simulink model "harmonic_tracker"  (R2025b)
settings: Solver=VariableStepAuto  StartTime=0.0  StopTime=1  RelTol=1e-3
values from neighbouring files (symbols this model uses):
  Ad_fht2 = eye(2) + Afht1*ts_inv + 1/2*Afht1^2*ts_inv^2    [init_model.m]
  Ad_fht3 = expm(Afht1*ts_inv)    [init_model.m]
  Cfht1 = [1 0]    [init_model.m]
  delta_fht1 = 0.05    [init_model.m]
  Ld_fht1 = acker(Ad_fht1',Cfht1', polesd_fht1)    [init_model.m]
  Ld_fht2 = acker(Ad_fht2',Cfht1', polesd_fht1)    [init_model.m]
  Ld_fht3 = acker(Ad_fht3',Cfht1', polesd_fht1)    [init_model.m]
  omega_fht1 = 2*pi*frequency_set    (= 2513.27412287)    [init_model.m]
  ts_afe = 1/fPWM_AFE    (= 0.0001)    [init_model.m]
  ts_inv = 1/fPWM_INV    (= 0.0001)    [init_model.m]
libraries: sogi_quadrature_generator_ccaller x1
settings Model: SimulationMode=accelerator  Creator=ltnbda  LastModifiedBy=dbagn
settings SFSimCC: SimCustomHeaderCode=|
  | #include "first_harmonic_tracker_simulink.h"
  | #include "first_harmonic_tracker.h"
  | #include "sogi_flt_simulink.h"
  | #include "sogi_flt.h"
  | #include "harmonic_tracker_simulink.h"
  | #include "harmonic_tracker.h"
settings SFSimCC: SimUserSources=|
  | "first_harmonic_tracker_simulink.c"
  | "first_harmonic_tracker.c"
  | "sogi_flt_simulink.c"
  | "sogi_flt.c"
  | "harmonic_tracker_simulink.c"
  | "harmonic_tracker.c"
settings SFSimCC: SimUserIncludeDirs=|
  | include
  | src

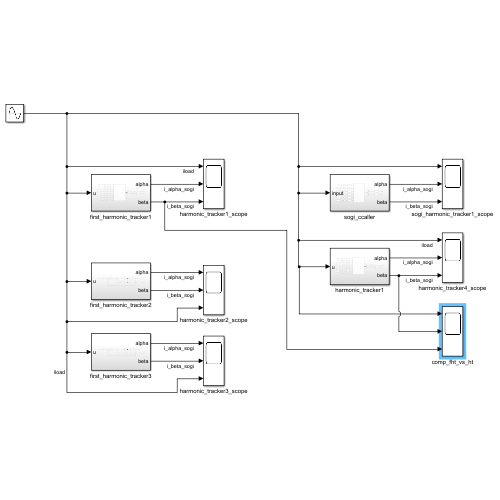
[thumbnail: Simulink's stored preview of the top-level diagram]
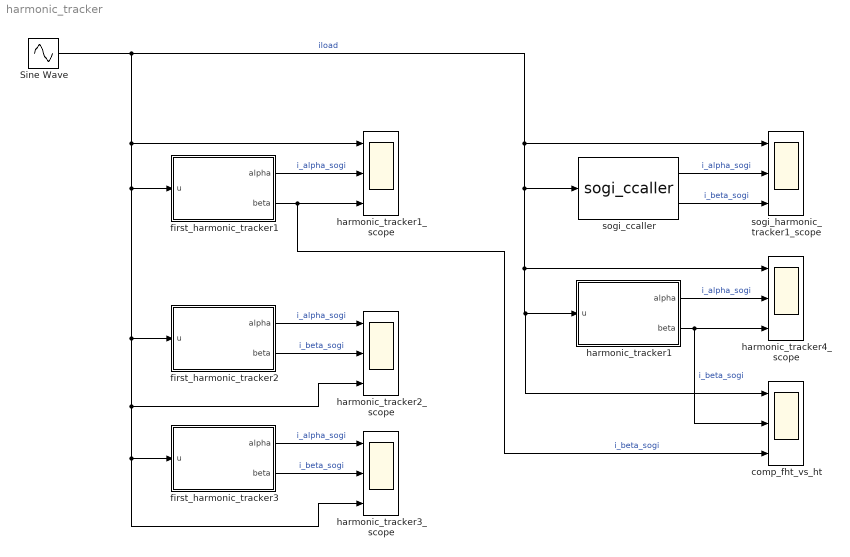
== system harmonic_tracker ==
  Sine Wave : Sin  Frequency=omega_fht1  SampleTime=0
  comp_fht_vs_ht : Scope  NumInputPorts=3
      settings: ActiveDisplayYMinimum=-1.6579339355230331  ActiveDisplayYMaximum=1.6235805600881577  DataLoggingVariableName=ScopeData5
  first_harmonic_tracker1 : Subsystem
  first_harmonic_tracker2 : Subsystem
  first_harmonic_tracker3 : Subsystem
  harmonic_tracker1 : Subsystem
  harmonic_tracker1_scope : Scope  NumInputPorts=3
      settings: ActiveDisplayYMinimum=-1.6579339355230331  ActiveDisplayYMaximum=1.6235805600881577
  harmonic_tracker2_scope : Scope  NumInputPorts=3
      settings: ActiveDisplayYMinimum=-1.2519895707446069  ActiveDisplayYMaximum=1.287638852418608
  harmonic_tracker3_scope : Scope  NumInputPorts=3
      settings: ActiveDisplayYMinimum=-1.251814205501226  ActiveDisplayYMaximum=1.2860605652281802  DataLoggingVariableName=ScopeData2
  harmonic_tracker4_scope : Scope  NumInputPorts=3
      settings: ActiveDisplayYMinimum=-1.6579339355230331  ActiveDisplayYMaximum=1.6235805600881577  DataLoggingVariableName=ScopeData4
  sogi_ccaller : sogi_quadrature_generator_ccaller/sogi_ccaller  SystemSampleTime=-1  VariantActivationTime=update diagram  EmptyChoice=off  PassThrough=off  PassThroughVariantControl=(default)  EmptyChoiceVariantControl=(default)  AllowFlexibleInterface=on  Latency=0  AutoFrameSizeCalculation=off
  sogi_harmonic_tracker1_scope : Scope  NumInputPorts=3
      settings: ActiveDisplayYMinimum=-1.4729834645986557  ActiveDisplayYMaximum=1.5802953094244003  DataLoggingVariableName=ScopeData3
  wires:
  first_harmonic_tracker1/1(alpha) -> harmonic_tracker1_scope/2  "i_alpha_sogi"
  first_harmonic_tracker1/2(beta) -> comp_fht_vs_ht/3, harmonic_tracker1_scope/3  "i_beta_sogi"
  first_harmonic_tracker2/1(alpha) -> harmonic_tracker2_scope/1  "i_alpha_sogi"
  first_harmonic_tracker2/2(beta) -> harmonic_tracker2_scope/2  "i_beta_sogi"
  first_harmonic_tracker3/2(beta) -> harmonic_tracker3_scope/2  "i_beta_sogi"
  first_harmonic_tracker3/1(alpha) -> harmonic_tracker3_scope/1  "i_alpha_sogi"
  sogi_ccaller/2 -> sogi_harmonic_tracker1_scope/3  "i_beta_sogi"
  sogi_ccaller/1 -> sogi_harmonic_tracker1_scope/2  "i_alpha_sogi"
  Sine Wave/1 -> sogi_ccaller/1, harmonic_tracker4_scope/1, comp_fht_vs_ht/1, harmonic_tracker1/1(u), sogi_harmonic_tracker1_scope/1, harmonic_tracker3_scope/3, first_harmonic_tracker3/1(u), harmonic_tracker2_scope/3, first_harmonic_tracker2/1(u), first_harmonic_tracker1/1(u), harmonic_tracker1_scope/1  "iload"
  harmonic_tracker1/2(beta) -> comp_fht_vs_ht/2, harmonic_tracker4_scope/3  "i_beta_sogi"
  harmonic_tracker1/1(alpha) -> harmonic_tracker4_scope/2  "i_alpha_sogi"

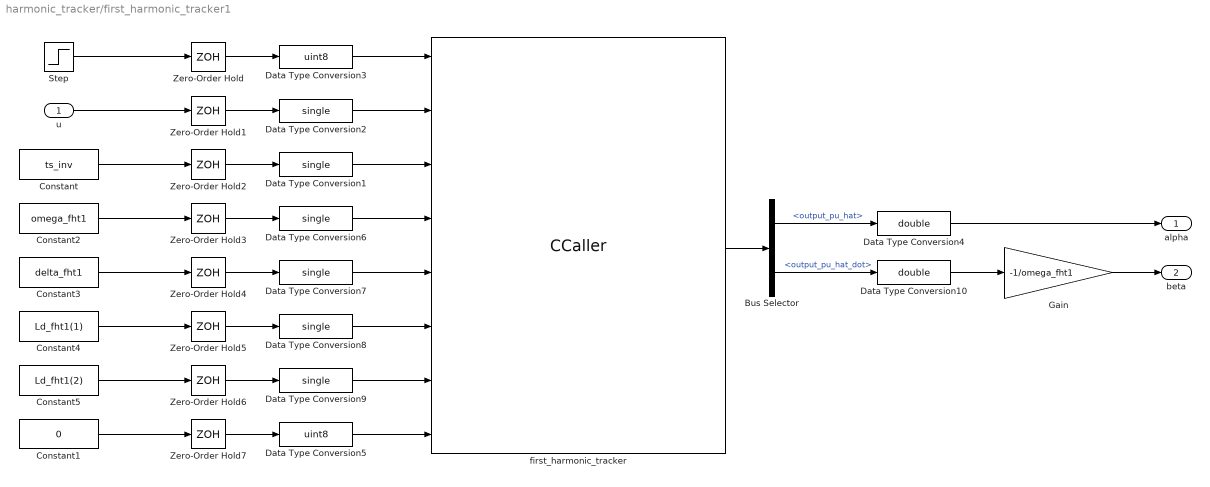
== system harmonic_tracker/first_harmonic_tracker1 ==
  u : Inport
  Bus Selector : BusSelector  OutputSignals=output_pu_hat,output_pu_hat_dot
  Constant : Constant  Value=ts_inv
  Constant1 : Constant  Value=0
  Constant2 : Constant  Value=omega_fht1
  Constant3 : Constant  Value=delta_fht1
  Constant4 : Constant  Value=Ld_fht1(1)
  Constant5 : Constant  Value=Ld_fht1(2)
  Data Type Conversion{1..2,6..9} (6 alike) : DataTypeConversion  OutDataTypeStr=single  SaturateOnIntegerOverflow=off  RndMeth=Floor
  Data Type Conversion10 : DataTypeConversion  OutDataTypeStr=double  SaturateOnIntegerOverflow=off  RndMeth=Floor
  Data Type Conversion3 : DataTypeConversion  OutDataTypeStr=uint8  SaturateOnIntegerOverflow=off  RndMeth=Floor
  Data Type Conversion4 : DataTypeConversion  OutDataTypeStr=double  SaturateOnIntegerOverflow=off  RndMeth=Floor
  Data Type Conversion5 : DataTypeConversion  OutDataTypeStr=uint8  SaturateOnIntegerOverflow=off  RndMeth=Floor
  Gain : Gain  Gain=-1/omega_fht1
  Step : Step  Time=0.0125  Before=1  After=0
  Zero-Order Hold{,1..7} (8 alike) : ZeroOrderHold  SampleTime=ts_inv
  first_harmonic_tracker : CCaller  FunctionName=first_harmonic_tracker_process_simulink  PortSpecificationStruct="%)30     .    B \\   8    (     @         %    \"     D    !     0         %  0 \"0    $    _    07)G3F%M90  4&]R=$YA;64 4V-O<&4     26YD97@     5'EP90      4VEZ90      27-';&]B86P   X    P    !@    @    $          4    (     0    ,    !         !   P!O=70 #@   #     &    \"     0         !0    @    !     P    $         $  # &]U=  .    .     8    (    !          %    \"     $    &     0         0  ...(+4988 chars)"  SampleTime=ts_inv
  alpha : Outport
  beta : Outport  Port=2
  wires:
  Data Type Conversion4/1 -> alpha/1
  Data Type Conversion3/1 -> first_harmonic_tracker/1
  Data Type Conversion1/1 -> first_harmonic_tracker/3
  Data Type Conversion2/1 -> first_harmonic_tracker/2
  first_harmonic_tracker/1 -> Bus Selector/1
  Bus Selector/1 -> Data Type Conversion4/1  "<output_pu_hat>"
  Step/1 -> Zero-Order Hold/1
  u/1 -> Zero-Order Hold1/1
  Constant/1 -> Zero-Order Hold2/1
  Constant1/1 -> Zero-Order Hold7/1
  Data Type Conversion5/1 -> first_harmonic_tracker/8
  Constant2/1 -> Zero-Order Hold3/1
  Data Type Conversion6/1 -> first_harmonic_tracker/4
  Constant3/1 -> Zero-Order Hold4/1
  Data Type Conversion7/1 -> first_harmonic_tracker/5
  Constant4/1 -> Zero-Order Hold5/1
  Data Type Conversion8/1 -> first_harmonic_tracker/6
  Constant5/1 -> Zero-Order Hold6/1
  Data Type Conversion9/1 -> first_harmonic_tracker/7
  Bus Selector/2 -> Data Type Conversion10/1  "<output_pu_hat_dot>"
  Data Type Conversion10/1 -> Gain/1
  Gain/1 -> beta/1
  Zero-Order Hold/1 -> Data Type Conversion3/1
  Zero-Order Hold1/1 -> Data Type Conversion2/1
  Zero-Order Hold2/1 -> Data Type Conversion1/1
  Zero-Order Hold3/1 -> Data Type Conversion6/1
  Zero-Order Hold4/1 -> Data Type Conversion7/1
  Zero-Order Hold5/1 -> Data Type Conversion8/1
  Zero-Order Hold6/1 -> Data Type Conversion9/1
  Zero-Order Hold7/1 -> Data Type Conversion5/1

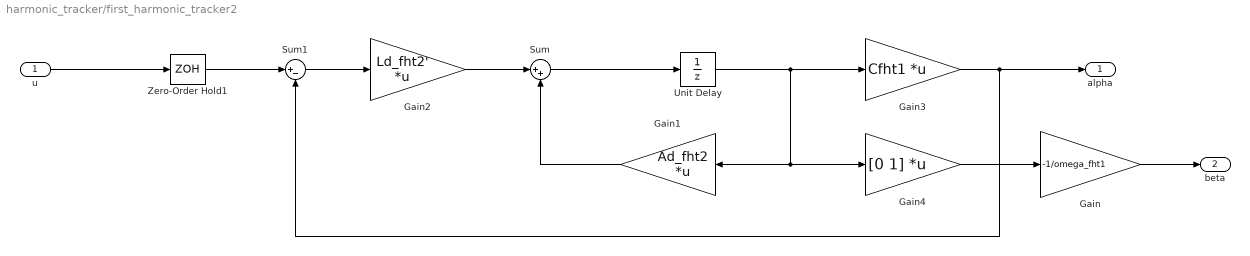
== system harmonic_tracker/first_harmonic_tracker2 ==
  u : Inport
  Gain : Gain  Gain=-1/omega_fht1
  Gain1 : Gain  Gain=Ad_fht2  Multiplication=Matrix(K*u)
  Gain2 : Gain  Gain=Ld_fht2'  Multiplication=Matrix(K*u)
  Gain3 : Gain  Gain=Cfht1  Multiplication=Matrix(K*u)
  Gain4 : Gain  Gain=[0 1]  Multiplication=Matrix(K*u)
  Sum : Sum  Inputs=|++
  Sum1 : Sum  Inputs=|+-
  Unit Delay : UnitDelay  SampleTime=ts_afe  HasFrameUpgradeWarning=on
  Zero-Order Hold1 : ZeroOrderHold  SampleTime=ts_inv
  alpha : Outport
  beta : Outport  Port=2
  wires:
  u/1 -> Zero-Order Hold1/1
  Sum/1 -> Unit Delay/1
  Unit Delay/1 -> Gain1/1, Gain4/1, Gain3/1
  Gain1/1 -> Sum/2
  Gain2/1 -> Sum/1
  Sum1/1 -> Gain2/1
  Zero-Order Hold1/1 -> Sum1/1
  Gain3/1 -> Sum1/2, alpha/1
  Gain4/1 -> Gain/1
  Gain/1 -> beta/1

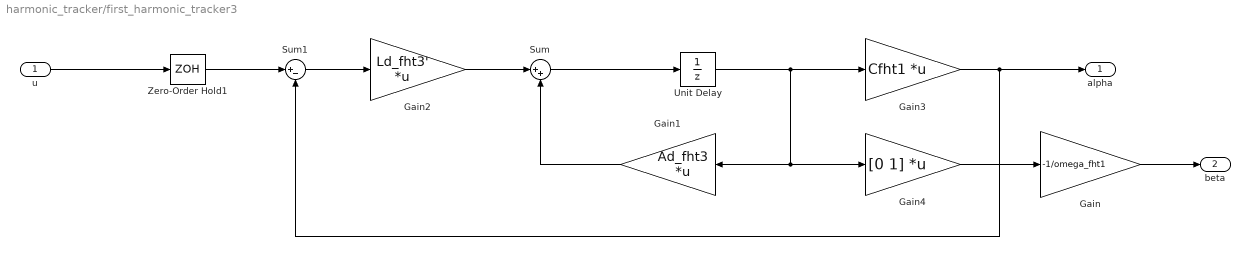
== system harmonic_tracker/first_harmonic_tracker3 ==
  u : Inport
  Gain : Gain  Gain=-1/omega_fht1
  Gain1 : Gain  Gain=Ad_fht3  Multiplication=Matrix(K*u)
  Gain2 : Gain  Gain=Ld_fht3'  Multiplication=Matrix(K*u)
  Gain3 : Gain  Gain=Cfht1  Multiplication=Matrix(K*u)
  Gain4 : Gain  Gain=[0 1]  Multiplication=Matrix(K*u)
  Sum : Sum  Inputs=|++
  Sum1 : Sum  Inputs=|+-
  Unit Delay : UnitDelay  SampleTime=ts_afe  HasFrameUpgradeWarning=on
  Zero-Order Hold1 : ZeroOrderHold  SampleTime=ts_inv
  alpha : Outport
  beta : Outport  Port=2
  wires:
  Gain/1 -> beta/1
  Gain4/1 -> Gain/1
  Gain3/1 -> alpha/1, Sum1/2
  Zero-Order Hold1/1 -> Sum1/1
  Sum1/1 -> Gain2/1
  Gain2/1 -> Sum/1
  Gain1/1 -> Sum/2
  Unit Delay/1 -> Gain3/1, Gain4/1, Gain1/1
  Sum/1 -> Unit Delay/1
  u/1 -> Zero-Order Hold1/1

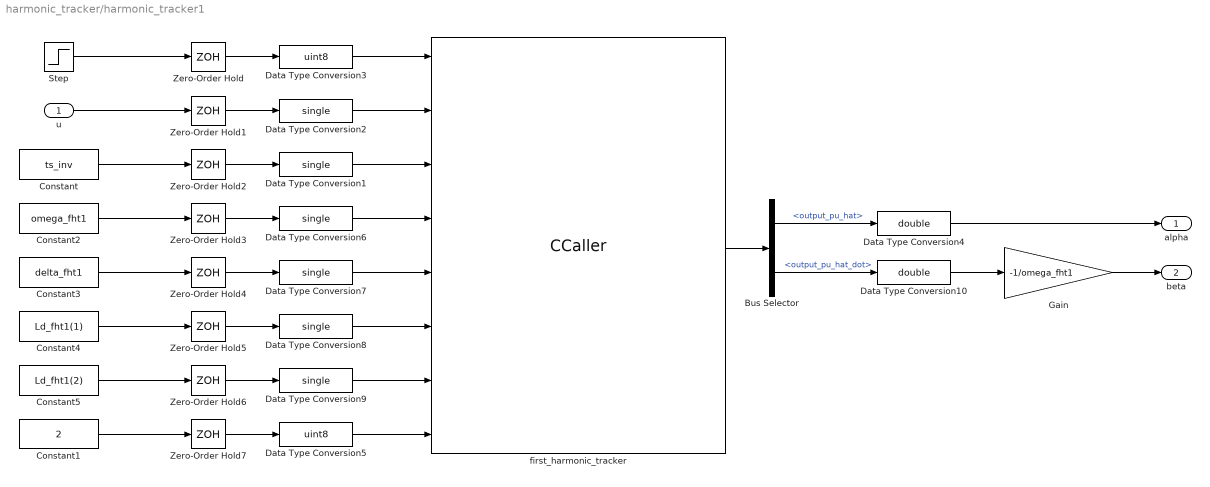
== system harmonic_tracker/harmonic_tracker1 ==
  u : Inport
  Bus Selector : BusSelector  OutputSignals=output_pu_hat,output_pu_hat_dot
  Constant : Constant  Value=ts_inv
  Constant1 : Constant  Value=2
  Constant2 : Constant  Value=omega_fht1
  Constant3 : Constant  Value=delta_fht1
  Constant4 : Constant  Value=Ld_fht1(1)
  Constant5 : Constant  Value=Ld_fht1(2)
  Data Type Conversion{1..2,6..9} (6 alike) : DataTypeConversion  OutDataTypeStr=single  SaturateOnIntegerOverflow=off  RndMeth=Floor
  Data Type Conversion10 : DataTypeConversion  OutDataTypeStr=double  SaturateOnIntegerOverflow=off  RndMeth=Floor
  Data Type Conversion3 : DataTypeConversion  OutDataTypeStr=uint8  SaturateOnIntegerOverflow=off  RndMeth=Floor
  Data Type Conversion4 : DataTypeConversion  OutDataTypeStr=double  SaturateOnIntegerOverflow=off  RndMeth=Floor
  Data Type Conversion5 : DataTypeConversion  OutDataTypeStr=uint8  SaturateOnIntegerOverflow=off  RndMeth=Floor
  Gain : Gain  Gain=-1/omega_fht1
  Step : Step  Time=0.0125  Before=1  After=0
  Zero-Order Hold{,1..7} (8 alike) : ZeroOrderHold  SampleTime=ts_inv
  first_harmonic_tracker : CCaller  FunctionName=harmonic_tracker_process_simulink  PortSpecificationStruct="%)30     .    @ \\   8    (     @         %    \"     D    !     0         %  0 \"0    $    _    07)G3F%M90  4&]R=$YA;64 4V-O<&4     26YD97@     5'EP90      4VEZ90      27-';&]B86P   X    P    !@    @    $          4    (     0    ,    !         !   P!O=70 #@   #     &    \"     0         !0    @    !     P    $         $  # &]U=  .    .     8    (    !          %    \"     $    &     0         0  ...(+4964 chars)"  SampleTime=ts_inv
  alpha : Outport
  beta : Outport  Port=2
  wires:
  Zero-Order Hold7/1 -> Data Type Conversion5/1
  Zero-Order Hold6/1 -> Data Type Conversion9/1
  Zero-Order Hold5/1 -> Data Type Conversion8/1
  Zero-Order Hold4/1 -> Data Type Conversion7/1
  Zero-Order Hold3/1 -> Data Type Conversion6/1
  Zero-Order Hold2/1 -> Data Type Conversion1/1
  Zero-Order Hold1/1 -> Data Type Conversion2/1
  Zero-Order Hold/1 -> Data Type Conversion3/1
  Gain/1 -> beta/1
  Data Type Conversion10/1 -> Gain/1
  Bus Selector/2 -> Data Type Conversion10/1  "<output_pu_hat_dot>"
  Data Type Conversion9/1 -> first_harmonic_tracker/7
  Constant5/1 -> Zero-Order Hold6/1
  Data Type Conversion8/1 -> first_harmonic_tracker/6
  Constant4/1 -> Zero-Order Hold5/1
  Data Type Conversion7/1 -> first_harmonic_tracker/5
  Constant3/1 -> Zero-Order Hold4/1
  Data Type Conversion6/1 -> first_harmonic_tracker/4
  Constant2/1 -> Zero-Order Hold3/1
  Data Type Conversion5/1 -> first_harmonic_tracker/8
  Constant1/1 -> Zero-Order Hold7/1
  Constant/1 -> Zero-Order Hold2/1
  u/1 -> Zero-Order Hold1/1
  Step/1 -> Zero-Order Hold/1
  Bus Selector/1 -> Data Type Conversion4/1  "<output_pu_hat>"
  first_harmonic_tracker/1 -> Bus Selector/1
  Data Type Conversion2/1 -> first_harmonic_tracker/2
  Data Type Conversion1/1 -> first_harmonic_tracker/3
  Data Type Conversion3/1 -> first_harmonic_tracker/1
  Data Type Conversion4/1 -> alpha/1
